simulink model "l1ac_ssc"  (R2016a)
settings: Solver=VariableStepAuto  StartTime=0.0  StopTime=10.0  MaxStep=1e-2  RelTol=1e-3
InitFcn:
  | configuration
StartFcn:
  | configuration
values from neighbouring files (symbols this model uses):
  Gamma = 10    [configuration.m]    (also in parameters.m = 1)
  kg = 1/(-C/A*B)    [configuration.m]
  knom = 2    [configuration.m]
  ref = 3    [configuration.m]
  sigma = 2    [configuration.m]    (also in parameters.m = 1)
  stepTimeRef = 1    [configuration.m]
  stepTimeSigma = 10    [configuration.m]
  tau_l1ac = 0.075    [configuration.m]
  tau_ssc = 0.001    [configuration.m]
  x0 = zeros(size(A,2),1)    [configuration.m]
  xm0 = zeros(size(Am,2),1)    [configuration.m]
undefined symbols (not defined in the file or in its folder): A, Am, B, Bm, C, Cm, D, Dm
settings Model: Creator=Gabriel-Lenovo  LastModifiedBy=Gabriel-Lenovo

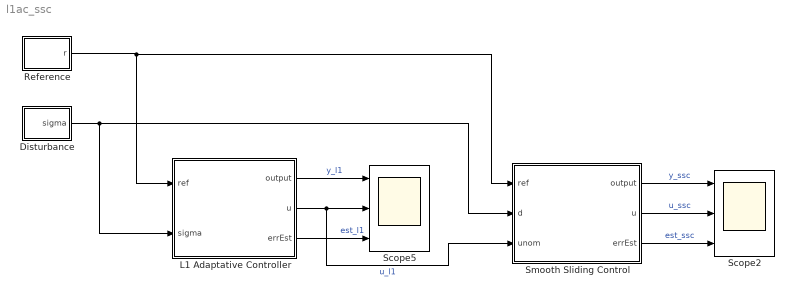
== system l1ac_ssc ==
  Disturbance : Subsystem
  L1 Adaptative Controller : Subsystem
  Reference : Subsystem
  Scope2 : Scope  NumInputPorts=3
  Scope5 : Scope  NumInputPorts=3
  Smooth Sliding Control : Subsystem
  wires:
  Disturbance/1(sigma) -> Smooth Sliding Control/2(d), L1 Adaptative Controller/2(sigma)
  L1 Adaptative Controller/1(output) -> Scope5/1  "y_l1"
  L1 Adaptative Controller/2(u) -> Smooth Sliding Control/3(unom), Scope5/2  "u_l1"
  L1 Adaptative Controller/3(errEst) -> Scope5/3  "est_l1"
  Smooth Sliding Control/1(output) -> Scope2/1  "y_ssc"
  Smooth Sliding Control/2(u) -> Scope2/2  "u_ssc"
  Smooth Sliding Control/3(errEst) -> Scope2/3  "est_ssc"
  Reference/1(r) -> Smooth Sliding Control/1(ref), L1 Adaptative Controller/1(ref)

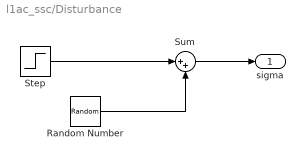
== system l1ac_ssc/Disturbance ==
  Random Number : RandomNumber  Variance=0
  Step : Step  Time=stepTimeSigma  After=sigma  SampleTime=0
  Sum : Sum  Inputs=|++
  sigma : Outport
  wires:
  Step/1 -> Sum/1
  Random Number/1 -> Sum/2
  Sum/1 -> sigma/1

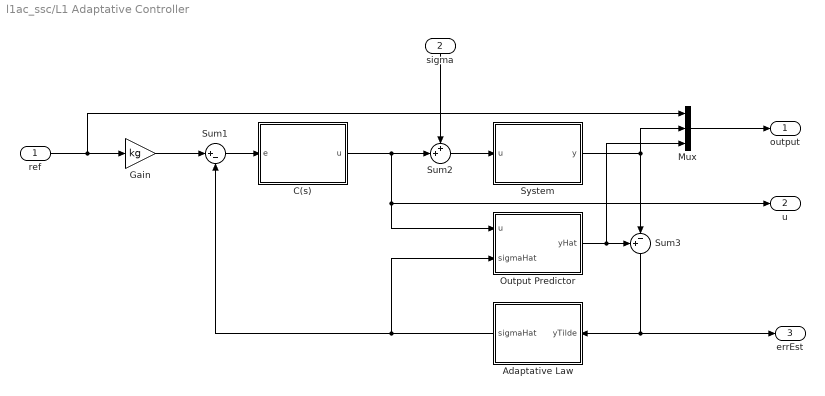
== system l1ac_ssc/L1 Adaptative Controller ==
  ref : Inport
  sigma : Inport  Port=2
  Adaptative Law : Subsystem
  C(s) : Subsystem
  Gain : Gain  Gain=kg
  Mux : Mux  Inputs=3
  Output Predictor : Subsystem
  Sum1 : Sum  Inputs=|+-
  Sum2 : Sum  Inputs=++|
  Sum3 : Sum  Inputs=+-|
  System : Subsystem
  output : Outport
  u : Outport  Port=2
  errEst : Outport  Port=3
  wires:
  ref/1 -> Mux/1, Gain/1
  sigma/1 -> Sum2/1
  Gain/1 -> Sum1/1
  Sum1/1 -> C(s)/1(e)
  Adaptative Law/1(sigmaHat) -> Sum1/2, Output Predictor/2(sigmaHat)
  Output Predictor/1(yHat) -> Mux/3, Sum3/1
  Sum2/1 -> System/1(u)
  Mux/1 -> output/1
  C(s)/1(u) -> Output Predictor/1("u "), u/1, Sum2/2
  Sum3/1 -> errEst/1, Adaptative Law/1(yTilde)
  System/1(y) -> Mux/2, Sum3/2

== system l1ac_ssc/Reference ==
  Step : Step  Time=stepTimeRef  After=ref  SampleTime=0
  r : Outport
  wires:
  Step/1 -> r/1

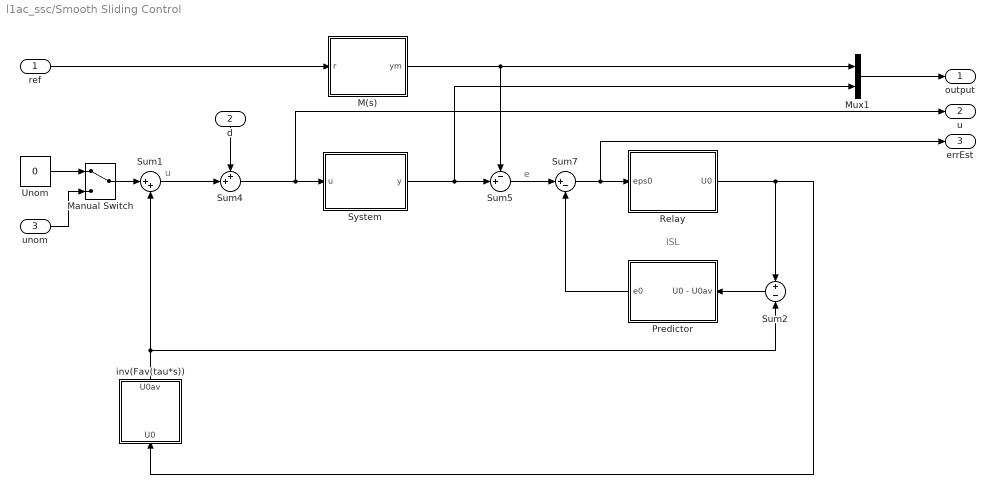
== system l1ac_ssc/Smooth Sliding Control ==
  note: u
  note: e
  note: ISL
  ref : Inport
  d : Inport  Port=2
  unom : Inport  Port=3
  M(s) : Subsystem
  Manual Switch : ManualSwitch
  Mux1 : Mux  Inputs=2
  Predictor : Subsystem
  Relay : Subsystem
  Sum1 : Sum  Inputs=|++
  Sum2 : Sum  Inputs=+|-
  Sum4 : Sum  Inputs=++|
  Sum5 : Sum  Inputs=-+|
  Sum7 : Sum  Inputs=|+-
  System : Subsystem
  Unom : Constant  Value=0
  inv(Fav(tau*s)) : Subsystem
  output : Outport
  u : Outport  Port=2
  errEst : Outport  Port=3
  wires:
  inv(Fav(tau*s))/1(U0av) -> Sum1/2, Sum2/2
  Sum7/1 -> errEst/1, Relay/1(eps0)
  Predictor/1(e0) -> Sum7/2
  System/1(y) -> Mux1/2, Sum5/2
  Relay/1(U0) -> Sum2/1, inv(Fav(tau*s))/1(U0)
  M(s)/1(ym) -> Sum5/1, Mux1/1
  Sum5/1 -> Sum7/1
  Sum4/1 -> u/1, System/1(u)
  Mux1/1 -> output/1
  ref/1 -> M(s)/1(r)
  d/1 -> Sum4/1
  Sum2/1 -> Predictor/1("U0 - U0av ")
  Sum1/1 -> Sum4/2
  Unom/1 -> Manual Switch/1
  unom/1 -> Manual Switch/2
  Manual Switch/1 -> Sum1/1

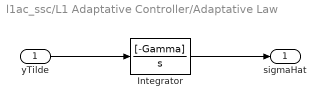
== system l1ac_ssc/L1 Adaptative Controller/Adaptative Law ==
  yTilde : Inport
  Integrator : TransferFcn  Numerator=[-Gamma]  Denominator=[1 0]
  sigmaHat : Outport
  wires:
  yTilde/1 -> Integrator/1
  Integrator/1 -> sigmaHat/1

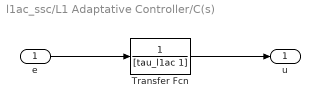
== system l1ac_ssc/L1 Adaptative Controller/C(s) ==
  e : Inport
  Transfer Fcn : TransferFcn  Denominator=[tau_l1ac 1]
  u : Outport
  wires:
  e/1 -> Transfer Fcn/1
  Transfer Fcn/1 -> u/1

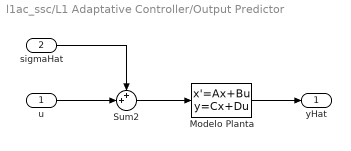
== system l1ac_ssc/L1 Adaptative Controller/Output Predictor ==
  "u " : Inport
  sigmaHat : Inport  Port=2
  Modelo Planta : StateSpace  A=A  B=B  C=C  D=D  X0=x0
  Sum2 : Sum  Inputs=++|
  yHat : Outport
  wires:
  Modelo Planta/1 -> yHat/1
  "u "/1 -> Sum2/2
  sigmaHat/1 -> Sum2/1
  Sum2/1 -> Modelo Planta/1

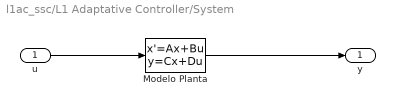
== system l1ac_ssc/L1 Adaptative Controller/System ==
  u : Inport
  Modelo Planta : StateSpace  A=A  B=B  C=C  D=D  X0=x0
  y : Outport
  wires:
  u/1 -> Modelo Planta/1
  Modelo Planta/1 -> y/1

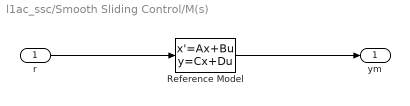
== system l1ac_ssc/Smooth Sliding Control/M(s) ==
  r : Inport
  Reference Model : StateSpace  A=Am  B=Bm  C=Cm  D=Dm  X0=xm0
  ym : Outport
  wires:
  r/1 -> Reference Model/1
  Reference Model/1 -> ym/1

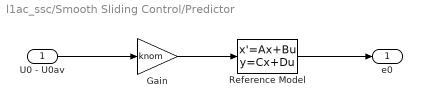
== system l1ac_ssc/Smooth Sliding Control/Predictor ==
  "U0 - U0av " : Inport
  Gain : Gain  Gain=knom
  Reference Model : StateSpace  A=Am  B=Bm  C=Cm  D=Dm  X0=xm0
  e0 : Outport
  wires:
  Reference Model/1 -> e0/1
  "U0 - U0av "/1 -> Gain/1
  Gain/1 -> Reference Model/1

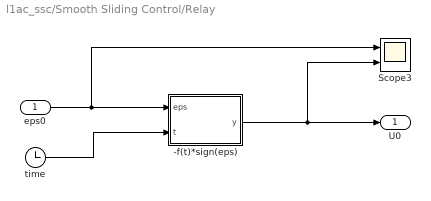
== system l1ac_ssc/Smooth Sliding Control/Relay ==
  eps0 : Inport
  -f(t)*sign(eps) : MATLAB Function  TreatAsAtomicUnit=on
  Scope3 : Scope  NumInputPorts=2
  time : Clock
  U0 : Outport
  wires:
  eps0/1 -> Scope3/1, -f(t)*sign(eps)/1(eps)
  -f(t)*sign(eps)/1(y) -> U0/1, Scope3/2
  time/1 -> -f(t)*sign(eps)/2(t)

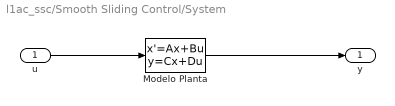
== system l1ac_ssc/Smooth Sliding Control/System ==
  u : Inport
  Modelo Planta : StateSpace  A=A  B=B  C=C  D=D  X0=x0
  y : Outport
  wires:
  u/1 -> Modelo Planta/1
  Modelo Planta/1 -> y/1

== system l1ac_ssc/Smooth Sliding Control/inv(Fav(tau*s)) ==
  U0 : Inport
  Fav^-1 : TransferFcn  Denominator=[tau_ssc 1]
  U0av : Outport
  wires:
  U0/1 -> Fav^-1/1
  Fav^-1/1 -> U0av/1

== matlab function l1ac_ssc/Smooth Sliding Control/Relay/-f(t)*sign(eps) ==
  data: eps input; y output; t input
function y = fcn(eps,t)
%#codegen
y = -modulation(t)*sign(eps);
